simulink model "sim_simulink"  (R2022a)
settings: Solver=VariableStepAuto  StartTime=0.0  StopTime=0.000005  RelTol=1e-3
undefined symbols (not defined in the file): a, b, c
libraries: msbPllFoundation x5, msbPllArchitectures x1, hdlsllib x1, cstblocks x1
settings Model: Creator=Herman  LastModifiedBy=Herman

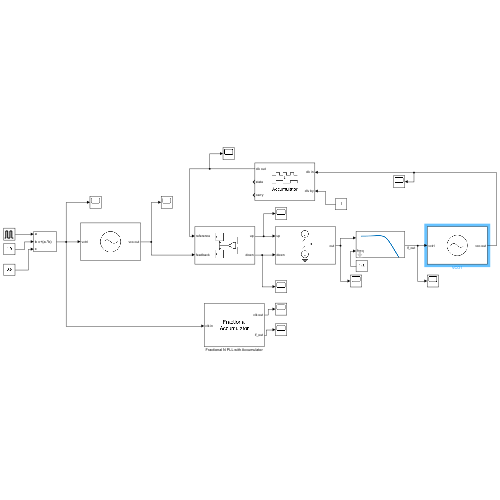
[thumbnail: Simulink's stored preview of the top-level diagram]
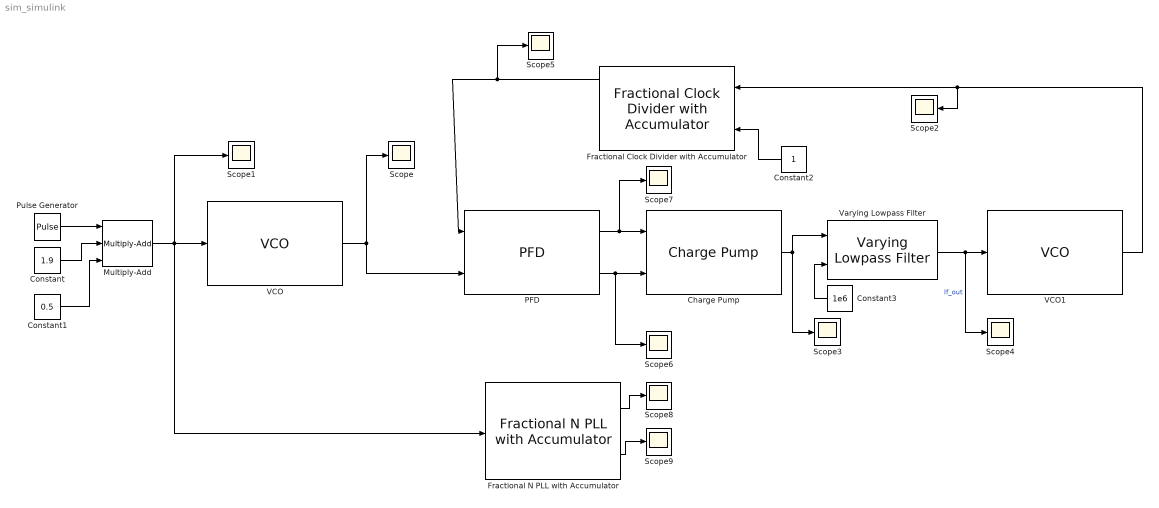
== system sim_simulink ==
  Charge Pump : msbPllFoundation/Charge Pump  OutputCurrent=1e-3  InputThreshold=0.5  ExtraBuffer=off  NBuffer=10  EnableCurrentImpairments=off  CurrentImbalance=1e-7  LeakageCurrent=1e-8  EnableTimingImpairments=off  DefaultOrAdvanced=Default  MaxFreqInterest=10e9  RiseFallUp=5e-9  PropDelayUp=6e-9  RiseFallDown=2e-9  PropDelayDown=4e-9
      settings: SourceProductBaseCode=AM
  Constant : Constant  Value=1.9
  Constant1 : Constant  Value=0.5
  Constant2 : Constant
  Constant3 : Constant  Value=1e6
  Fractional Clock Divider with Accumulator : msbPllFoundation/Fractional Clock Divider with Accumulator  ExtraBuffer=off  NBuffer=1
      settings: SourceProductBaseCode=AM
  Fractional N PLL with Accumulator : msbPllArchitectures/Fractional N PLL with Accumulator  DeadbandCompensation=40e-12  EnableImpairments=off  DefaultOrAdvanced=Default  MaxFreqInterest=10e9  RiseFallTime=3e-11  PropDelay=50e-12  OutputCurrent=1e-3  InputThreshold=0.5  EnableCurrentImpairments=off  CurrentImbalance=1e-7  LeakageCurrent=1e-8  EnableTimingImpairments=off  MaxFreqInterestCp=10e9  DefaultOrAdvancedCp=Default  RiseFallUp=5e-9  PropDelayUp=6e-9  RiseFallDown=2e-9  PropDelayDown=4e-9  SpecifyUsing=Voltage sensitivity  Kvco=100e6  ControlVoltage=[-5 0 5]  OutputFrequency=[2e9 2.5e9 3e9]  MaxKvco=100000000  Fo=1.8e9  Amplitude=1  AddPhaseNoise=off  Foffset=[30e3 100e3 1e6 3e6 10e6]  PhaseNoise=[-56 -106 -132 -143 -152]  N=70.20  Nmin=70  CompSelectionMethod=Automatic  Fc=0.5e6  Phi=45  FilterType="3rd  order passive"  C1=3e-11  C2=3.3e-10  C3=2.15e-12  C4=1e-12  R2=2.33e+03  R3=2.98e+04  R4=12e3  LfEnableImpairments=off  Temperature=30  pfd_up_dn=off  cp_out=off  lf_out=on  ps_out=off  ol_opt=on  cl_opt=off  ExtraBuffer=off  NBufferFilter=1000  NBuffer=10
      settings: SourceProductBaseCode=AM
  Multiply-Add : hdlsllib/HDL Operations/Multiply-Add  Function=c+(a.*b)  datatype=Inherit: Inherit via internal rule  DoSatur=off  FMA=off
      settings: SourceProductBaseCode=SL
  PFD : msbPllFoundation/PFD  DeadbandCompensation=30e-12  ExtraBuffer=off  NBuffer=10  EnableImpairments=off  DefaultOrAdvanced=Default  MaxFreqInterest=10e9  RiseFallTime=30e-12  PropDelay=50e-12
      settings: SourceProductBaseCode=AM
  Pulse Generator : DiscretePulseGenerator  PulseType=Time based  Period=3e-8  PulseWidth=50
  Scope{,1..9} (10 alike) : Scope
  VCO : msbPllFoundation/VCO  SpecifyUsing=Voltage sensitivity  Kvco=100e6  Fo=1200e6  ControlVoltage=[0.5 1.4 2.5]  OutputFrequency=[2e9 2.5e9 3e9]  Amplitude=1  ExtraBuffer=off  NBuffer=10  AddPhaseNoise=off  Foffset=[30e3 100e3 1e6 3e6 10e6]  PhaseNoise=[-56 -106 -132 -143 -152]  MaxKvco=100000000
      settings: SourceProductBaseCode=AM
  VCO1 : msbPllFoundation/VCO  SpecifyUsing=Output frequency vs. control voltage  Kvco=100e6  Fo=1200e6  ControlVoltage=[0.5 1.4 2.5]  OutputFrequency=[1145e6 1200e6 1250e6]  Amplitude=1  ExtraBuffer=off  NBuffer=10  AddPhaseNoise=off  Foffset=[30e3 100e3 1e6 3e6 10e6]  PhaseNoise=[-56 -106 -132 -143 -152]  MaxKvco=61111111.1111
      settings: SourceProductBaseCode=AM
  Varying Lowpass Filter : cstblocks/Linear Parameter Varying/Varying Lowpass Filter  N=1
  wires:
  Multiply-Add/1 -> Fractional N PLL with Accumulator/1, VCO/1, Scope1/1
  Pulse Generator/1 -> Multiply-Add/1
  Constant/1 -> Multiply-Add/2
  Constant1/1 -> Multiply-Add/3
  VCO/1 -> PFD/2, Scope/1
  PFD/1 -> Scope7/1, Charge Pump/1
  PFD/2 -> Scope6/1, Charge Pump/2
  Constant2/1 -> Fractional Clock Divider with Accumulator/2
  Fractional Clock Divider with Accumulator/1 -> Scope5/1, PFD/1
  Charge Pump/1 -> Varying Lowpass Filter/1, Scope3/1
  Varying Lowpass Filter/1 -> Scope4/1, VCO1/1  "lf_out"
  VCO1/1 -> Fractional Clock Divider with Accumulator/1, Scope2/1
  Constant3/1 -> Varying Lowpass Filter/2
  Fractional N PLL with Accumulator/1 -> Scope8/1
  Fractional N PLL with Accumulator/2 -> Scope9/1
